simulink model "momentumObserver"  (R2020a)
settings: Solver=VariableStepAuto  StartTime=0.0  StopTime=nrOfSamples  FixedStep=0.001  RelTol=1e-3
undefined symbols (not defined in the file): F_ext, nrOfJoints
settings Model: Creator=iiticublap041  LastModifiedBy=iiticublap041
settings SolverCC: ZeroCrossAlgorithm=Adaptive
settings DataIOCC: ExternalInput=dataset

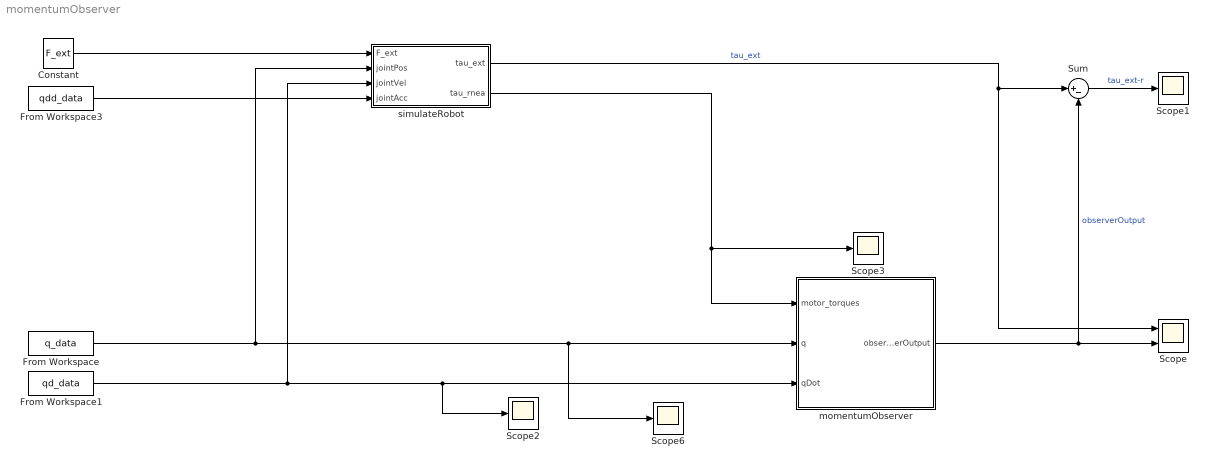
== system momentumObserver ==
  Constant : Constant  Value=F_ext
  From Workspace : FromWorkspace  VariableName=q_data
  From Workspace1 : FromWorkspace  VariableName=qd_data
  From Workspace3 : FromWorkspace  VariableName=qdd_data
  Scope : Scope  NumInputPorts=2
  Scope{1..3,6} (4 alike) : Scope
  Sum : Sum  Inputs=|+-
  momentumObserver : Subsystem
  simulateRobot : Subsystem
  wires:
  From Workspace/1 -> simulateRobot/2(jointPos), momentumObserver/2(q), Scope6/1
  momentumObserver/1(observerOutput) -> Sum/2, Scope/2  "observerOutput"
  From Workspace1/1 -> simulateRobot/3(jointVel), momentumObserver/3(qDot), Scope2/1
  Sum/1 -> Scope1/1  "tau_ext-r"
  simulateRobot/1(tau_ext) -> Scope/1, Sum/1  "tau_ext"
  simulateRobot/2(tau_rnea) -> Scope3/1, momentumObserver/1(motor_torques)
  Constant/1 -> simulateRobot/1(F_ext)
  From Workspace3/1 -> simulateRobot/4(jointAcc)

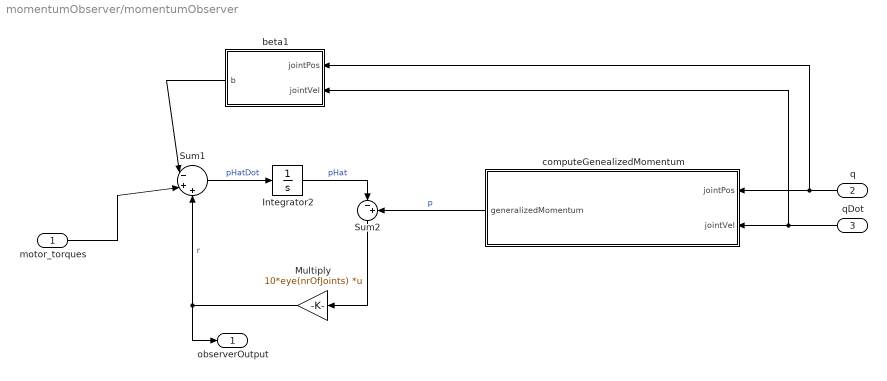
== system momentumObserver/momentumObserver ==
  motor_torques : Inport
  q : Inport  Port=2
  qDot : Inport  Port=3
  Integrator2 : Integrator
  Multiply : Gain  Gain=10*eye(nrOfJoints)  Multiplication=Matrix(K*u) (u vector)
  Sum1 : Sum  Inputs=|-++
  Sum2 : Sum  Inputs=|-+
  beta1 : MATLAB Function  TreatAsAtomicUnit=on
  computeGenealizedMomentum : MATLAB Function  TreatAsAtomicUnit=on
  observerOutput : Outport
  wires:
  Sum1/1 -> Integrator2/1  "pHatDot"
  Multiply/1 -> Sum1/3, observerOutput/1  "r"
  computeGenealizedMomentum/1(generalizedMomentum) -> Sum2/2  "p"
  beta1/1(b) -> Sum1/1
  Sum2/1 -> Multiply/1
  Integrator2/1 -> Sum2/1  "pHat"
  motor_torques/1 -> Sum1/2
  qDot/1 -> beta1/2(jointVel), computeGenealizedMomentum/2(jointVel)
  q/1 -> computeGenealizedMomentum/1(jointPos), beta1/1(jointPos)

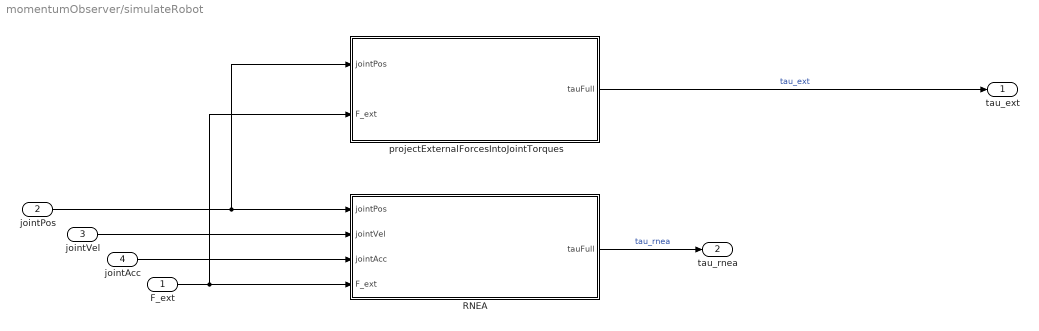
== system momentumObserver/simulateRobot ==
  F_ext : Inport
  jointPos : Inport  Port=2
  jointVel : Inport  Port=3
  jointAcc : Inport  Port=4
  RNEA : MATLAB Function  TreatAsAtomicUnit=on
  projectExternalForcesIntoJointTorques : MATLAB Function  TreatAsAtomicUnit=on
  tau_ext : Outport
  tau_rnea : Outport  Port=2
  wires:
  jointVel/1 -> RNEA/2(jointVel)
  projectExternalForcesIntoJointTorques/1(tauFull) -> tau_ext/1  "tau_ext"
  F_ext/1 -> projectExternalForcesIntoJointTorques/2(F_ext), RNEA/4(F_ext)
  jointPos/1 -> projectExternalForcesIntoJointTorques/1(jointPos), RNEA/1(jointPos)
  RNEA/1(tauFull) -> tau_rnea/1  "tau_rnea"
  jointAcc/1 -> RNEA/3(jointAcc)

== matlab function momentumObserver/simulateRobot/projectExternalForcesIntoJointTorques ==
  data: jointPos input; tauFull output; F_ext input
function tauFull = projectExternalForcesIntoJointTorques(jointPos,F_ext)

% Use rnea mex function
coder.extrinsic('computeNumericalJacobian');
J = computeNumericalJacobian('computeNumericalJacobian',jointPos);
% Assign the output to a vaiable of known type.
% See https://www.mathworks.com/help/simulink/ug/calling-matlab-functions.html#bq1h2z9-47
tauFull = zeros(max(size(jointPos)),1);
tauFull = full(J).'*F_ext(:,end);
end

== matlab function momentumObserver/beta1 ==
  data: jointPos input; b output; jointVel input
function b = beta(jointPos,jointVel)
% Compute gravity torques using RNEA with appropriate inputs
qd_grav = 0;
qdd = 0;
F_ext = 0;
% TODO: do not hard code gravity 
g = [0;0;-9.81];
coder.extrinsic('rnea');
tau_gravity = rnea('rnea',jointPos,qd_grav,qdd,g,F_ext);
% Assign the output to a vaiable of kwown type.
% See https://www.mathworks.com/help/simulink/ug/calling-matlab-functions.html#bq1h2z9-47
tau_gravityFull = zeros(max(size(jointPos,1)),1);
tau_gravityFull = full(tau_gravity);
% Coriolis matrix
coder.extrinsic('computeCoriolisMatrix');
C = computeCoriolisMatrix('computeCoriolisMatrix',jointPos,jointVel);
CFull = zeros(max(size(jointPos,1)));
CFull = full(C);
b = tau_gravityFull - CFull.'*jointVel;

== matlab function momentumObserver/computeGenealizedMomentum ==
  data: jointPos input; jointVel input; generalizedMomentum output
function generalizedMomentum = computeGeneralizedMomentum(jointPos,jointVel)
coder.extrinsic('computeMassMatrix'); 
M = computeMassMatrix('computeMassMatrix', jointPos);
% Assign the output to a vaiable of kwown type.
% See https://www.mathworks.com/help/simulink/ug/calling-matlab-functions.html#bq1h2z9-47
MFull = zeros(max(size(jointPos)));
MFull = full(M);
generalizedMomentum = MFull*jointVel;

== matlab function momentumObserver/simulateRobot/RNEA ==
  data: jointPos input; jointVel input; tauFull output; jointAcc input; F_ext input
function tauFull = RNEA(jointPos,jointVel,jointAcc,F_ext)

% TODO: do not hard code gravity 
g = [0;0;-9.81];
% Use rnea mex function
coder.extrinsic('rnea');
tau = rnea('rnea',jointPos,jointVel,jointAcc,g,F_ext);
% Assign the output to a vaiable of known type.
% See https://www.mathworks.com/help/simulink/ug/calling-matlab-functions.html#bq1h2z9-47
tauFull = zeros(max(size(jointPos)),1);
tauFull = full(tau);
end
